simulink model "windrad_PID"  (R2020a)
settings: Solver=ode45  StartTime=0.0  StopTime=200  FixedStep=1e-4  RelTol=1e-9
values from neighbouring files (symbols this model uses):
  a = 0.0158    [windrad_init.m]
  b = 0.00084    [windrad_init.m]
  c = 0.0127    [windrad_init.m]
  k = 11.5    [windrad_init.m]
  Kp = b/a    (= 0.053164556962)    [windrad_init.m]
  T1 = 1/a    (= 63.2911392405)    [windrad_init.m]
  T_PID = 0.002    [windrad_init.m]
  Tt = 0.2    [windrad_init.m]
settings Model: Creator=Ravi Plenzdorf  LastModifiedBy=seife
settings DataIOCC: ReturnWorkspaceOutputs=off

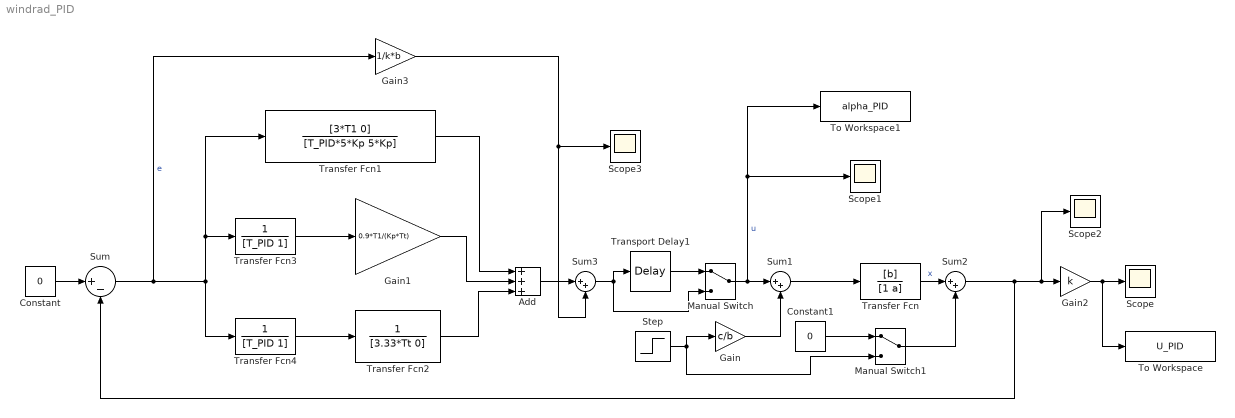
== system windrad_PID ==
  Add : Sum  Inputs=+++
  Constant : Constant  Value=0
  Constant1 : Constant  Value=0
  Gain : Gain  Gain=c/b
  Gain1 : Gain  Gain=0.9*T1/(Kp*Tt)
  Gain2 : Gain  Gain=k
  Gain3 : Gain  Gain=1/k*b
  Manual Switch : ManualSwitch
  Manual Switch1 : ManualSwitch
  Scope{,1..3} (4 alike) : Scope
  Step : Step  Time=2  SampleTime=0
  Sum : Sum  Inputs=|+-
  Sum1 : Sum  Inputs=|++
  Sum2 : Sum  Inputs=|++
  Sum3 : Sum  Inputs=|++
  To Workspace : ToWorkspace  VariableName=U_PID  SaveFormat=Timeseries  SampleTime=-1
  To Workspace1 : ToWorkspace  VariableName=alpha_PID  SaveFormat=Timeseries  SampleTime=-1
  Transfer Fcn : TransferFcn  Numerator=[b]  Denominator=[1 a]
  Transfer Fcn1 : TransferFcn  Numerator=[3*T1 0]  Denominator=[T_PID*5*Kp 5*Kp]
  Transfer Fcn2 : TransferFcn  Denominator=[3.33*Tt 0]
  Transfer Fcn3 : TransferFcn  Denominator=[T_PID 1]
  Transfer Fcn4 : TransferFcn  Denominator=[T_PID 1]
  Transport Delay1 : TransportDelay  DelayTime=Tt
  wires:
  Constant1/1 -> Manual Switch1/1
  Sum2/1 -> Sum/2, Scope2/1, Gain2/1
  Transfer Fcn/1 -> Sum2/1  "x"
  Constant/1 -> Sum/1
  Manual Switch1/1 -> Sum2/2
  Manual Switch/1 -> To Workspace1/1, Scope1/1, Sum1/1  "u"
  Step/1 -> Manual Switch1/2, Gain/1
  Gain1/1 -> Add/2
  Gain/1 -> Sum1/2
  Sum1/1 -> Transfer Fcn/1
  Transport Delay1/1 -> Manual Switch/1
  Transfer Fcn2/1 -> Add/3
  Gain2/1 -> To Workspace/1, Scope/1
  Transfer Fcn1/1 -> Add/1
  Transfer Fcn3/1 -> Gain1/1
  Transfer Fcn4/1 -> Transfer Fcn2/1
  Sum/1 -> Gain3/1, Transfer Fcn1/1, Transfer Fcn3/1, Transfer Fcn4/1  "e"
  Add/1 -> Sum3/1
  Sum3/1 -> Manual Switch/2, Transport Delay1/1
  Gain3/1 -> Scope3/1, Sum3/2
